simulink model "ExampleNegativeVar"  (R2017b)
settings: Solver=VariableStepAuto  StartTime=0.0  StopTime=1000000000000000000.0  RelTol=1e-3
settings Model: Creator=aarrieta  LastModifiedBy=aarrieta

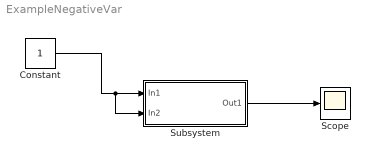
== system ExampleNegativeVar ==
  Constant : Constant
  Scope : Scope
  Subsystem : Subsystem
  wires:
  Constant/1 -> Subsystem/2(In2), Subsystem/1(In1)
  Subsystem/1(Out1) -> Scope/1

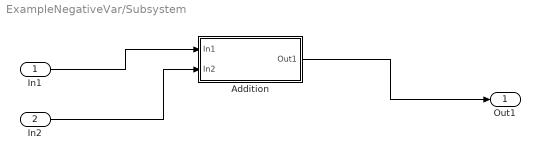
== system ExampleNegativeVar/Subsystem ==
  In1 : Inport
  In2 : Inport  Port=2
  Addition : Subsystem
  Out1 : Outport
  wires:
  In1/1 -> Addition/1(In1)
  In2/1 -> Addition/2(In2)
  Addition/1(Out1) -> Out1/1

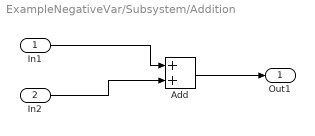
== system ExampleNegativeVar/Subsystem/Addition ==
  In1 : Inport
  In2 : Inport  Port=2
  Add : Sum
  Out1 : Outport
  wires:
  In1/1 -> Add/1
  In2/1 -> Add/2
  Add/1 -> Out1/1
